simulink model "homework_2_sim_dist_obs"  (R2018b)
settings: Solver=VariableStepAuto  StartTime=0.0  StopTime=15  MaxStep=1e-3  MinStep=1e-4  RelTol=1e-3
values from neighbouring files (symbols this model uses):
  A = A-B*K0    [homework_2_dist_obs.m]    (also in homework_2_local_obs.m)
  B = [0 -9.9453]'    [homework_2_dist_obs.m]    (also in homework_2_local_obs.m)
  c = 10*1/(2*min(real(lam_g)))    [homework_2_dist_obs.m]    (also in homework_2_local_obs.m = 5*1/(2*min(real(lam_g))))
  C = [708.27 0]    [homework_2_dist_obs.m]    (also in homework_2_local_obs.m)
  D = [0]    [homework_2_dist_obs.m]    (also in homework_2_local_obs.m)
  F = P*C'*R^-1    [homework_2_dist_obs.m]    (also in homework_2_local_obs.m = place(A', -c*C', [-10; -20])')
  G_ext = zeros(7, 7)    [homework_2_dist_obs.m]    (also in homework_2_local_obs.m)
  K = R^-1*B'*P    [homework_2_dist_obs.m]    (also in homework_2_local_obs.m)
  x0_f = [0.1818 0.1455; 0.8693 0.5499; 0.8530 0.3510;      0.2638 0.1361; 0.5797 0.1450; 0.6221 0.5132]'    [homework_2_dist_obs.m]    (also in homework_2_local_obs.m)
  x0_l = [1 1]    [homework_2_dist_obs.m]    (also in homework_2_local_obs.m)
libraries: simulink x6
settings Model: Creator=franc  LastModifiedBy=mluser
settings SolverCC: MaxConsecutiveMinStep=50
settings DataIOCC: ReturnWorkspaceOutputs=on

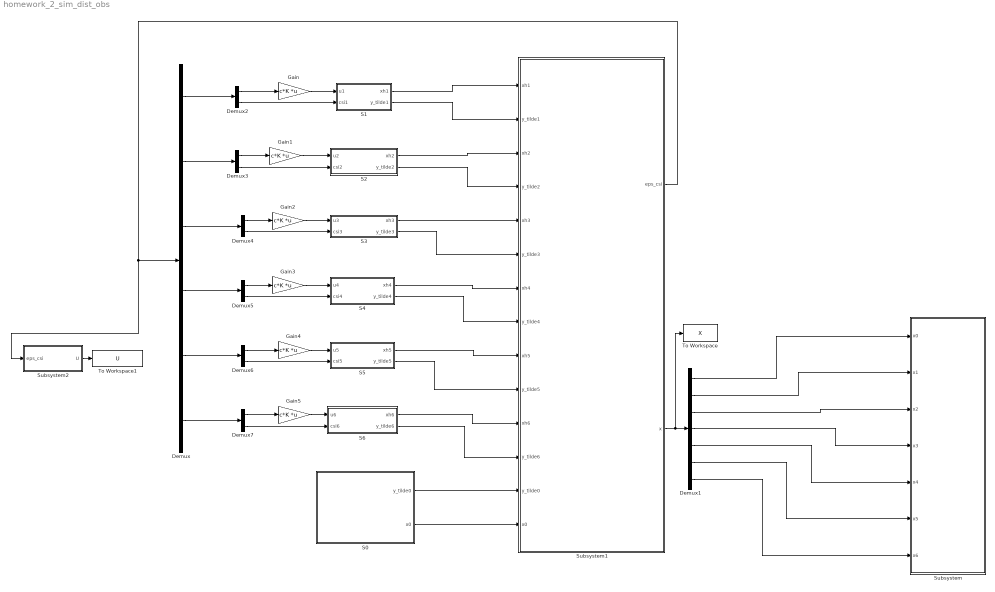
== system homework_2_sim_dist_obs ==
  Demux : Demux  Outputs=6
  Demux1 : Demux  Outputs=7
  Demux{2..7} (6 alike) : Demux  Outputs=2
  Gain{,1..5} (6 alike) : Gain  Gain=c*K  Multiplication=Matrix(K*u)
  S0 : Subsystem
  S1 : Subsystem
  S2 : Subsystem
  S3 : Subsystem
  S4 : Subsystem
  S5 : Subsystem
  S6 : Subsystem
  Subsystem : Subsystem
  Subsystem1 : Subsystem
  Subsystem2 : Subsystem
  To Workspace : ToWorkspace  VariableName=X  SaveFormat=Timeseries  SampleTime=-1
  To Workspace1 : ToWorkspace  VariableName=U  SaveFormat=Timeseries  SampleTime=-1
  wires:
  Demux1/5 -> Subsystem/5(x4)
  S2/1(xh2) -> Subsystem1/3(xh2)
  S0/2(x0) -> Subsystem1/14(x0)
  S2/2(y_tilde2) -> Subsystem1/4(y_tilde2)
  S4/2(y_tilde4) -> Subsystem1/8(y_tilde4)
  S3/2(y_tilde3) -> Subsystem1/6(y_tilde3)
  S6/2(y_tilde6) -> Subsystem1/12(y_tilde6)
  S1/2(y_tilde1) -> Subsystem1/2(y_tilde1)
  S6/1(xh6) -> Subsystem1/11(xh6)
  S5/2(y_tilde5) -> Subsystem1/10(y_tilde5)
  Demux1/2 -> Subsystem/2(x1)
  S0/1(y_tilde0) -> Subsystem1/13(y_tilde0)
  Demux1/4 -> Subsystem/4(x3)
  S1/1(xh1) -> Subsystem1/1(xh1)
  Demux1/3 -> Subsystem/3(x2)
  S3/1(xh3) -> Subsystem1/5(xh3)
  S4/1(xh4) -> Subsystem1/7(xh4)
  Subsystem1/2(x) -> To Workspace/1, Demux1/1
  S5/1(xh5) -> Subsystem1/9(xh5)
  Demux1/7 -> Subsystem/7(x6)
  Demux1/1 -> Subsystem/1(x0)
  Demux1/6 -> Subsystem/6(x5)
  Subsystem1/1(eps_csi) -> Subsystem2/1(eps_csi), Demux/1
  Demux/1 -> Demux2/1
  Demux2/1 -> Gain/1
  Gain/1 -> S1/1(u1)
  Demux2/2 -> S1/2(csi1)
  Demux3/1 -> Gain1/1
  Demux3/2 -> S2/2(csi2)
  Gain1/1 -> S2/1(u2)
  Demux/2 -> Demux3/1
  Demux4/1 -> Gain2/1
  Gain2/1 -> S3/1(u3)
  Demux4/2 -> S3/2(csi3)
  Demux/3 -> Demux4/1
  Demux/6 -> Demux7/1
  Demux/4 -> Demux5/1
  Demux/5 -> Demux6/1
  Demux5/1 -> Gain3/1
  Demux5/2 -> S4/2(csi4)
  Gain3/1 -> S4/1(u4)
  Demux6/1 -> Gain4/1
  Demux6/2 -> S5/2(csi5)
  Gain4/1 -> S5/1(u5)
  Demux7/1 -> Gain5/1
  Gain5/1 -> S6/1(u6)
  Demux7/2 -> S6/2(csi6)
  Subsystem2/1(U) -> To Workspace1/1

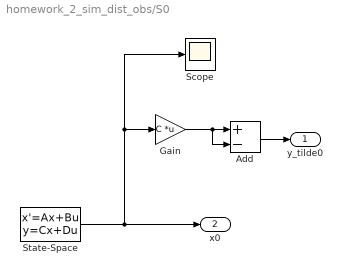
== system homework_2_sim_dist_obs/S0 ==
  Add : Sum  Inputs=+-
  Gain : Gain  Gain=C  Multiplication=Matrix(K*u)
  Scope : Scope
  State-Space : StateSpace  A=A  B=B  C=eye(2)  D=zeros(2,1)  InitialCondition=x0_l
  y_tilde0 : Outport
  x0 : Outport  Port=2
  wires:
  State-Space/1 -> Scope/1, Gain/1, x0/1
  Add/1 -> y_tilde0/1
  Gain/1 -> Add/2, Add/1

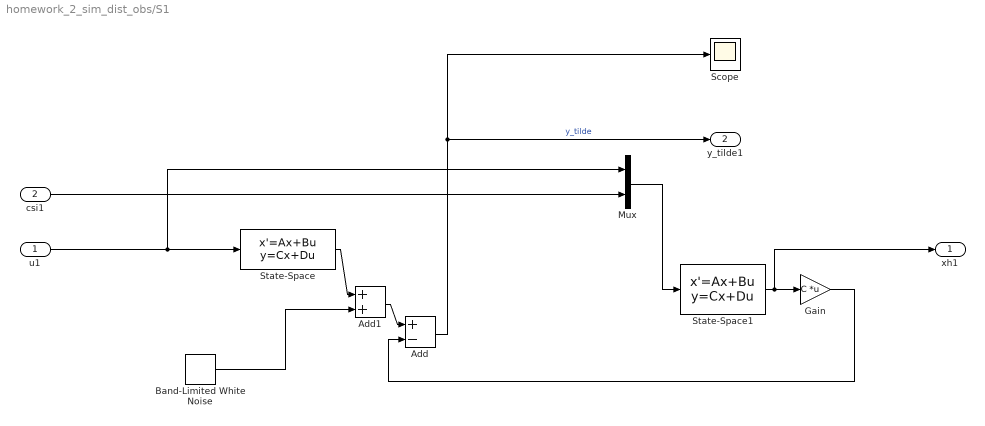
== system homework_2_sim_dist_obs/S1 ==
  u1 : Inport
  csi1 : Inport  Port=2  PortDimensions=1
  Add : Sum  Inputs=+-
  Add1 : Sum
  Band-Limited White Noise : simulink/Sources/Band-Limited White Noise  Cov=n  Ts=0.1  seed=[23341]
  Gain : Gain  Gain=C  Multiplication=Matrix(K*u)
  Mux : Mux  Inputs=2
  Scope : Scope
  State-Space : StateSpace  A=A  B=B  C=C  D=D  InitialCondition=x0_f(:,1)
  State-Space1 : StateSpace  A=A  B=[B -c*F]  C=eye(2)  D=[zeros(2, 1) zeros(2,1)]  InitialCondition=0
  xh1 : Outport
  y_tilde1 : Outport  Port=2
  wires:
  u1/1 -> Mux/1, State-Space/1
  Mux/1 -> State-Space1/1
  Gain/1 -> Add/2
  State-Space1/1 -> xh1/1, Gain/1
  Add/1 -> y_tilde1/1, Scope/1  "y_tilde"
  csi1/1 -> Mux/2
  State-Space/1 -> Add1/1
  Add1/1 -> Add/1
  Band-Limited White Noise/1 -> Add1/2

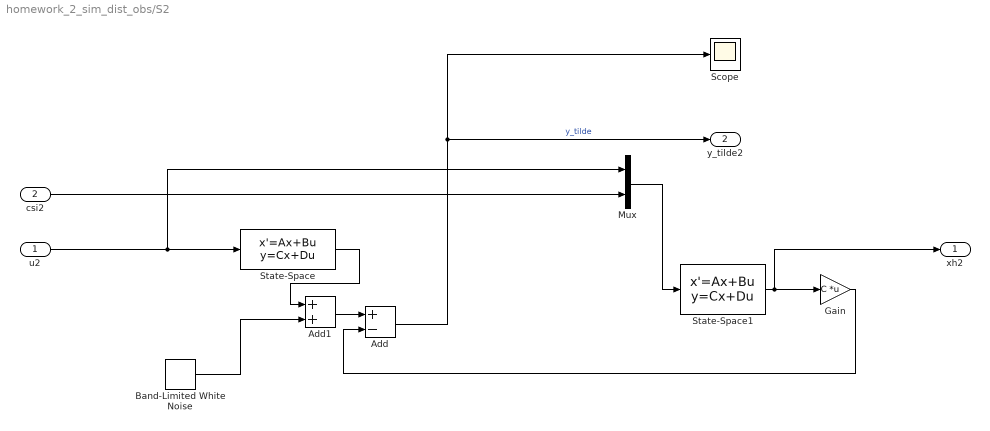
== system homework_2_sim_dist_obs/S2 ==
  u2 : Inport
  csi2 : Inport  Port=2  PortDimensions=1
  Add : Sum  Inputs=+-
  Add1 : Sum
  Band-Limited White Noise : simulink/Sources/Band-Limited White Noise  Cov=n  Ts=0.1  seed=[23441]
  Gain : Gain  Gain=C  Multiplication=Matrix(K*u)
  Mux : Mux  Inputs=2
  Scope : Scope
  State-Space : StateSpace  A=A  B=B  C=C  D=D  InitialCondition=x0_f(:,2)
  State-Space1 : StateSpace  A=A  B=[B -c*F]  C=eye(2)  D=[zeros(2, 1) zeros(2,1)]  InitialCondition=0
  xh2 : Outport
  y_tilde2 : Outport  Port=2
  wires:
  State-Space1/1 -> xh2/1, Gain/1
  Gain/1 -> Add/2
  u2/1 -> Mux/1, State-Space/1
  Add/1 -> y_tilde2/1, Scope/1  "y_tilde"
  Mux/1 -> State-Space1/1
  csi2/1 -> Mux/2
  Add1/1 -> Add/1
  State-Space/1 -> Add1/1
  Band-Limited White Noise/1 -> Add1/2

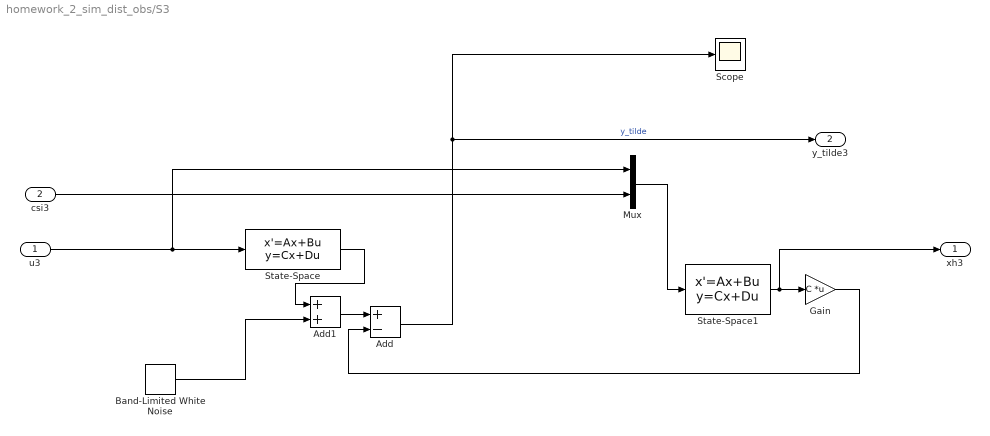
== system homework_2_sim_dist_obs/S3 ==
  u3 : Inport
  csi3 : Inport  Port=2  PortDimensions=1
  Add : Sum  Inputs=+-
  Add1 : Sum
  Band-Limited White Noise : simulink/Sources/Band-Limited White Noise  Cov=n  Ts=0.1  seed=[23541]
  Gain : Gain  Gain=C  Multiplication=Matrix(K*u)
  Mux : Mux  Inputs=2
  Scope : Scope
  State-Space : StateSpace  A=A  B=B  C=C  D=D  InitialCondition=x0_f(:,3)
  State-Space1 : StateSpace  A=A  B=[B -c*F]  C=eye(2)  D=[zeros(2, 1) zeros(2,1)]  InitialCondition=0
  xh3 : Outport
  y_tilde3 : Outport  Port=2
  wires:
  State-Space1/1 -> xh3/1, Gain/1
  u3/1 -> Mux/1, State-Space/1
  Mux/1 -> State-Space1/1
  Gain/1 -> Add/2
  Add/1 -> Scope/1, y_tilde3/1  "y_tilde"
  csi3/1 -> Mux/2
  Add1/1 -> Add/1
  State-Space/1 -> Add1/1
  Band-Limited White Noise/1 -> Add1/2

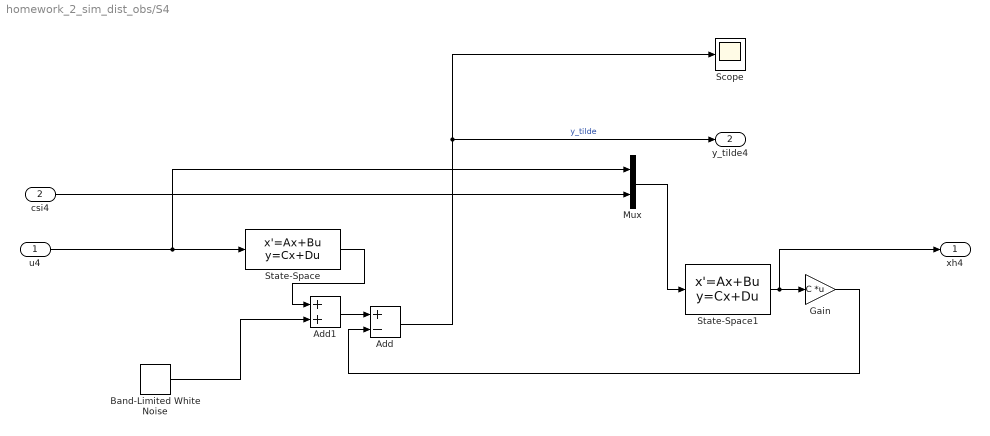
== system homework_2_sim_dist_obs/S4 ==
  u4 : Inport
  csi4 : Inport  Port=2  PortDimensions=1
  Add : Sum  Inputs=+-
  Add1 : Sum
  Band-Limited White Noise : simulink/Sources/Band-Limited White Noise  Cov=n  Ts=0.1  seed=[23641]
  Gain : Gain  Gain=C  Multiplication=Matrix(K*u)
  Mux : Mux  Inputs=2
  Scope : Scope
  State-Space : StateSpace  A=A  B=B  C=C  D=D  InitialCondition=x0_f(:,4)
  State-Space1 : StateSpace  A=A  B=[B -c*F]  C=eye(2)  D=[zeros(2, 1) zeros(2,1)]  InitialCondition=0
  xh4 : Outport
  y_tilde4 : Outport  Port=2
  wires:
  State-Space1/1 -> xh4/1, Gain/1
  u4/1 -> Mux/1, State-Space/1
  Mux/1 -> State-Space1/1
  Gain/1 -> Add/2
  Add/1 -> y_tilde4/1, Scope/1  "y_tilde"
  csi4/1 -> Mux/2
  Add1/1 -> Add/1
  State-Space/1 -> Add1/1
  Band-Limited White Noise/1 -> Add1/2

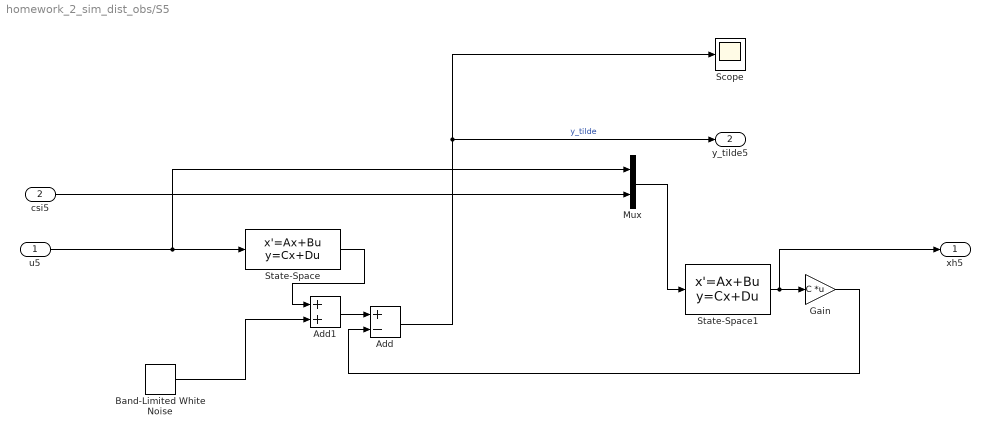
== system homework_2_sim_dist_obs/S5 ==
  u5 : Inport
  csi5 : Inport  Port=2  PortDimensions=1
  Add : Sum  Inputs=+-
  Add1 : Sum
  Band-Limited White Noise : simulink/Sources/Band-Limited White Noise  Cov=n  Ts=0.1  seed=[23741]
  Gain : Gain  Gain=C  Multiplication=Matrix(K*u)
  Mux : Mux  Inputs=2
  Scope : Scope
  State-Space : StateSpace  A=A  B=B  C=C  D=D  InitialCondition=x0_f(:,5)
  State-Space1 : StateSpace  A=A  B=[B -c*F]  C=eye(2)  D=[zeros(2, 1) zeros(2,1)]  InitialCondition=0
  xh5 : Outport
  y_tilde5 : Outport  Port=2
  wires:
  State-Space1/1 -> xh5/1, Gain/1
  u5/1 -> Mux/1, State-Space/1
  Mux/1 -> State-Space1/1
  Gain/1 -> Add/2
  Add/1 -> y_tilde5/1, Scope/1  "y_tilde"
  csi5/1 -> Mux/2
  Add1/1 -> Add/1
  State-Space/1 -> Add1/1
  Band-Limited White Noise/1 -> Add1/2

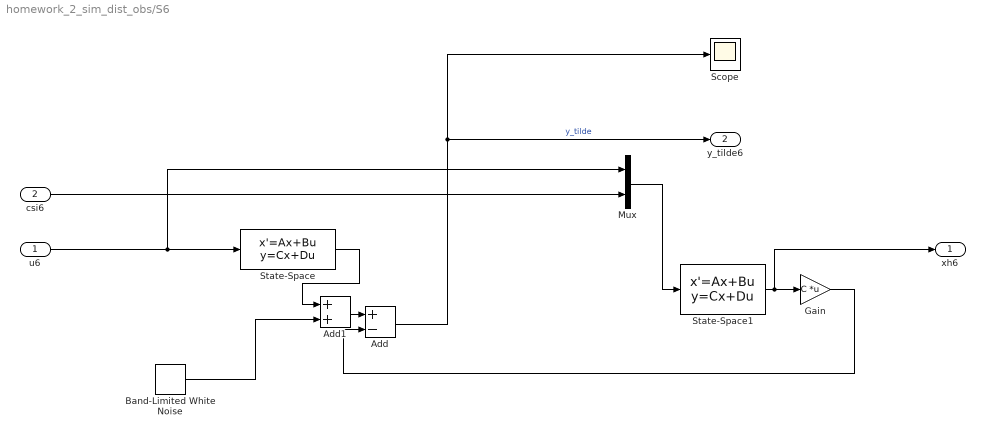
== system homework_2_sim_dist_obs/S6 ==
  u6 : Inport
  csi6 : Inport  Port=2  PortDimensions=1
  Add : Sum  Inputs=+-
  Add1 : Sum
  Band-Limited White Noise : simulink/Sources/Band-Limited White Noise  Cov=n  Ts=0.1  seed=[23841]
  Gain : Gain  Gain=C  Multiplication=Matrix(K*u)
  Mux : Mux  Inputs=2
  Scope : Scope
  State-Space : StateSpace  A=A  B=B  C=C  D=D  InitialCondition=x0_f(:,6)
  State-Space1 : StateSpace  A=A  B=[B -c*F]  C=eye(2)  D=[zeros(2, 1) zeros(2,1)]  InitialCondition=0
  xh6 : Outport
  y_tilde6 : Outport  Port=2
  wires:
  State-Space1/1 -> xh6/1, Gain/1
  u6/1 -> Mux/1, State-Space/1
  Mux/1 -> State-Space1/1
  Gain/1 -> Add/2
  Add/1 -> y_tilde6/1, Scope/1  "y_tilde"
  csi6/1 -> Mux/2
  Add1/1 -> Add/1
  State-Space/1 -> Add1/1
  Band-Limited White Noise/1 -> Add1/2

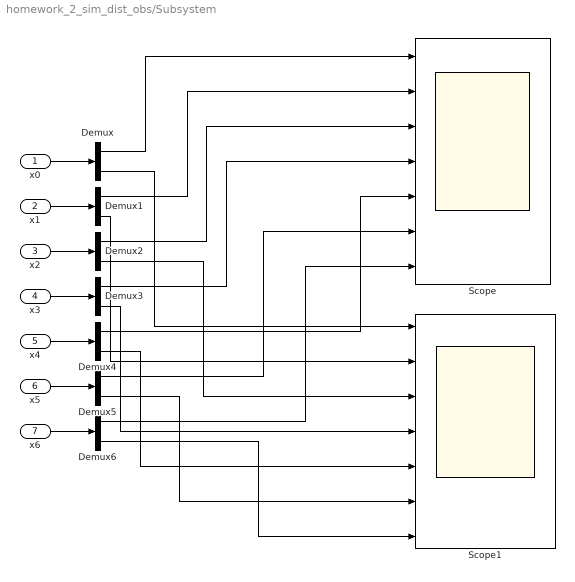
== system homework_2_sim_dist_obs/Subsystem ==
  x0 : Inport
  x1 : Inport  Port=2
  x2 : Inport  Port=3
  x3 : Inport  Port=4
  x4 : Inport  Port=5
  x5 : Inport  Port=6
  x6 : Inport  Port=7
  Demux{,1..6} (7 alike) : Demux  Outputs=2
  Scope : Scope  NumInputPorts=7
  Scope1 : Scope  NumInputPorts=7
  wires:
  x0/1 -> Demux/1
  x6/1 -> Demux6/1
  x5/1 -> Demux5/1
  x4/1 -> Demux4/1
  x3/1 -> Demux3/1
  x2/1 -> Demux2/1
  x1/1 -> Demux1/1
  Demux/1 -> Scope/1
  Demux1/1 -> Scope/2
  Demux2/1 -> Scope/3
  Demux3/1 -> Scope/4
  Demux5/1 -> Scope/6
  Demux6/1 -> Scope/7
  Demux/2 -> Scope1/1
  Demux1/2 -> Scope1/2
  Demux2/2 -> Scope1/3
  Demux4/1 -> Scope/5
  Demux3/2 -> Scope1/4
  Demux4/2 -> Scope1/5
  Demux5/2 -> Scope1/6
  Demux6/2 -> Scope1/7

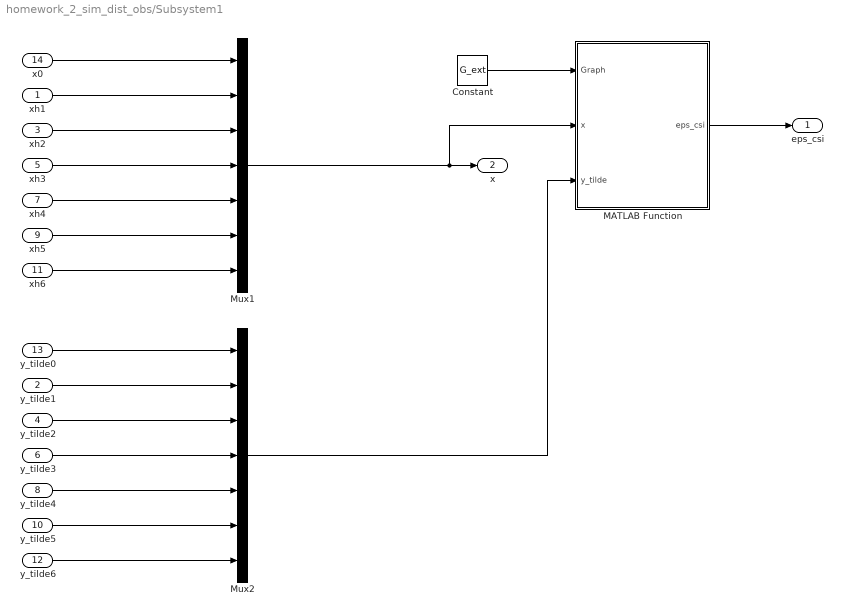
== system homework_2_sim_dist_obs/Subsystem1 ==
  xh1 : Inport
  y_tilde1 : Inport  Port=2
  xh2 : Inport  Port=3
  y_tilde2 : Inport  Port=4
  xh3 : Inport  Port=5
  y_tilde3 : Inport  Port=6
  xh4 : Inport  Port=7
  y_tilde4 : Inport  Port=8
  xh5 : Inport  Port=9
  y_tilde5 : Inport  Port=10
  xh6 : Inport  Port=11
  y_tilde6 : Inport  Port=12
  y_tilde0 : Inport  Port=13
  x0 : Inport  Port=14
  Constant : Constant  Value=G_ext
  MATLAB Function : MATLAB Function  TreatAsAtomicUnit=on
  Mux1 : Mux  Inputs=7
  Mux2 : Mux  Inputs=7
  eps_csi : Outport
  x : Outport  Port=2
  wires:
  Mux1/1 -> x/1, MATLAB Function/2(x)
  Constant/1 -> MATLAB Function/1(Graph)
  MATLAB Function/1(eps_csi) -> eps_csi/1
  xh6/1 -> Mux1/7
  xh5/1 -> Mux1/6
  xh4/1 -> Mux1/5
  xh3/1 -> Mux1/4
  xh2/1 -> Mux1/3
  xh1/1 -> Mux1/2
  x0/1 -> Mux1/1
  y_tilde4/1 -> Mux2/5
  y_tilde5/1 -> Mux2/6
  y_tilde6/1 -> Mux2/7
  y_tilde1/1 -> Mux2/2
  y_tilde2/1 -> Mux2/3
  y_tilde3/1 -> Mux2/4
  y_tilde0/1 -> Mux2/1
  Mux2/1 -> MATLAB Function/3(y_tilde)

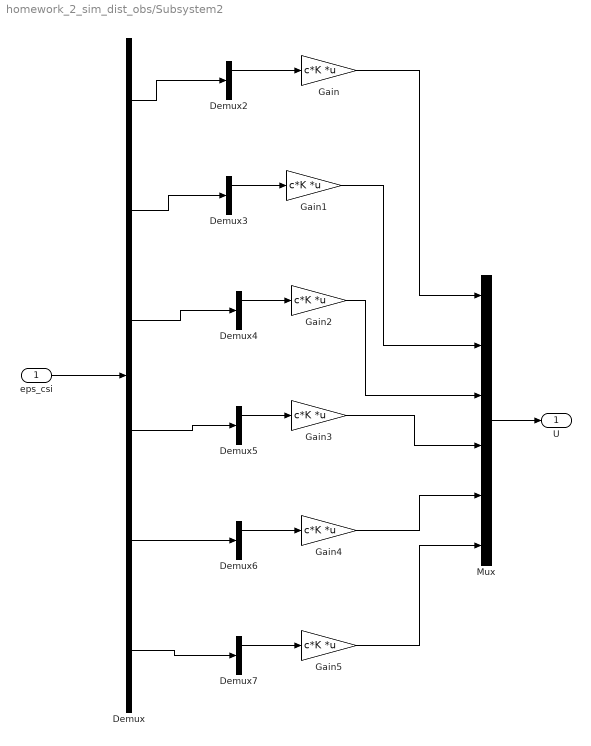
== system homework_2_sim_dist_obs/Subsystem2 ==
  eps_csi : Inport
  Demux : Demux  Outputs=6
  Demux{2..7} (6 alike) : Demux  Outputs=2
  Gain{,1..5} (6 alike) : Gain  Gain=c*K  Multiplication=Matrix(K*u)
  Mux : Mux  Inputs=6
  U : Outport
  wires:
  eps_csi/1 -> Demux/1
  Demux4/1 -> Gain2/1
  Demux/2 -> Demux3/1
  Demux/4 -> Demux5/1
  Demux5/1 -> Gain3/1
  Demux/1 -> Demux2/1
  Demux3/1 -> Gain1/1
  Demux7/1 -> Gain5/1
  Demux/6 -> Demux7/1
  Demux/3 -> Demux4/1
  Demux2/1 -> Gain/1
  Demux/5 -> Demux6/1
  Demux6/1 -> Gain4/1
  Mux/1 -> U/1
  Gain/1 -> Mux/1
  Gain1/1 -> Mux/2
  Gain2/1 -> Mux/3
  Gain3/1 -> Mux/4
  Gain4/1 -> Mux/5
  Gain5/1 -> Mux/6

== matlab function homework_2_sim_dist_obs/Subsystem1/MATLAB Function ==
  data: Graph input; eps_csi output; x input; y_tilde input
function eps_csi = fcn(Graph, x, y_tilde)

tmp = zeros(3,6);%colonne del tipo [eps1(i),eps2(i),csi(i)]'

x0=x(1:2);
x=reshape(x(3:end), 2, 6);
y_tilde0=y_tilde(1);
y_tilde=reshape(y_tilde(2:end), 1, 6);

Adj=Graph(2:end, 2:end);
G=Graph(2:end, 1);

for i=1:1:6 %calcolo eps per ogni nodo
    
    tmp(1:2,i) = G(i)*(x0-x(:,i));
    tmp(3,i) = G(i)*(y_tilde0-y_tilde(i));
    
    %contributo altri nodi
    for j = 1:6 
        tmp(1:2,i) = tmp(1:2,i) + Adj(i, j)*(x(:,j)-x(:,i));
        tmp(3,i) = tmp(3,i) + Adj(i, j)*(y_tilde(j)-y_tilde(i));
    end
end

eps_csi = reshape(tmp,18,1);
end
